simulink model "scheme"  (R2020a)
settings: Solver=VariableStepAuto  StartTime=0.0  StopTime=100  RelTol=1e-3
values from neighbouring files (symbols this model uses):
  G1 = K_r_d.Numerator{1, 1}    [script.m]
  G2 = K_r_d.Denominator{1, 1}    [script.m]
  Ts_ = 0.1    [script.m]
libraries: simulink x1
settings Model: Creator=User  LastModifiedBy=User

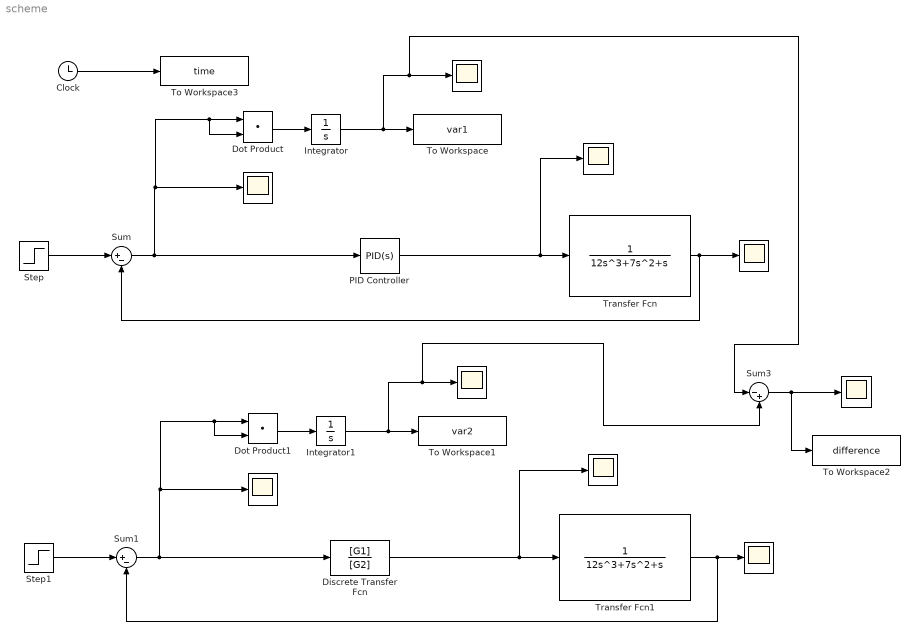
== system scheme ==
  " " : Scope
  "  " : Scope
  "   " : Scope
  "    " : Scope
  "     " : Scope
  "                 " : Scope
  "                       " : Scope
  "                                       " : Scope
  "                                                        " : Scope
  Clock : Clock
  Discrete Transfer Fcn : DiscreteTransferFcn  Numerator=[G1]  Denominator=[G2]  SampleTime=Ts_
  Dot Product : DotProduct  InputSameDT=on  OutDataTypeStr=Inherit: Inherit via internal rule
  Dot Product1 : DotProduct  InputSameDT=on  OutDataTypeStr=Inherit: Inherit via internal rule
  Integrator : Integrator
  Integrator1 : Integrator
  PID Controller : simulink/Continuous/PID Controller  Controller=PID  Form=Parallel  TimeDomain=Continuous-time  UseExternalTs=off  SampleTime=-1  IntegratorMethod=Forward Euler  FilterMethod=Forward Euler  ControllerParametersSource=internal  P=0.2897  I=0.006773  D=2.007  UseFilter=on  N=35.18  TunerSelectOption=Transfer Function Based (PID Tuner App)  InitialConditionSource=internal  InitialConditionForIntegrator=0  InitialConditionForFilter=0  DifferentiatorICPrevScaledInput=0  ExternalReset=none  TrackingMode=off  Kt=1  LimitOutput=off  UpperSaturationLimit=inf  LowerSaturationLimit=-inf  LinearizeAsGain=on  AntiWindupMode=none  Kb=1  POutMin=[]  POutMax=[]  IOutMin=[]  IOutMax=[]  DOutMin=[]  DOutMax=[]  NOutMin=[]  NOutMax=[]  SumOutMin=[]  SumOutMax=[]  SaturationOutMin=[]  SaturationOutMax=[]  PParamMin=[]  PParamMax=[]  IParamMin=[]  IParamMax=[]  DParamMin=[]  DParamMax=[]  NParamMin=[]  NParamMax=[]  KbParamMin=[]  KbParamMax=[]  KtParamMin=[]  KtParamMax=[]  KbOutMin=[]  KbOutMax=[]  KtOutMin=[]  KtOutMax=[]  IntegratorOutMin=[]  IntegratorOutMax=[]  FilterOutMin=[]  FilterOutMax=[]  SumI1OutMin=[]  SumI1OutMax=[]  SumI2OutMin=[]  SumI2OutMax=[]  SumI3OutMin=[]  SumI3OutMax=[]  SumI4OutMin=[]  SumI4OutMax=[]  SumDOutMin=[]  SumDOutMax=[]  DifferentiatorOutMin=[]  DifferentiatorOutMax=[]  FilterDiffOutCoefMin=[]  FilterDiffOutCoefMax=[]  ReciprocalOutMin=[]  ReciprocalOutMax=[]  SumDenOutMin=[]  SumDenOutMax=[]  SumNumOutMin=[]  SumNumOutMax=[]  DivideOutMin=[]  DivideOutMax=[]  UdiffTsProdOutMin=[]  UdiffTsProdOutMax=[]  NTsProdOutMin=[]  NTsProdOutMax=[]  UintegralTsProdOutMin=[]  UintegralTsProdOutMax=[]  UngainTsProdOutMin=[]  UngainTsProdOutMax=[]  IntegratorContinuousStateAttributes=''  IntegratorStateMustResolveToSignalObject=off  IntegratorRTWStateStorageClass=Auto  FilterContinuousStateAttributes=''  FilterStateMustResolveToSignalObject=off  FilterRTWStateStorageClass=Auto  ParallelPVariant=InternalParameters  IdealPVariant=Disabled  IVariant=InternalParameters  DVariant=InternalParameters  IntegratorVariant=Continuous  SatVariant=Disabled  AWVariant=Passthrough  PCopyVariant=Disabled  TRVariant=Disabled  FdbkBlocksVariant=Forward  IdealPFdbkVariant=Disabled  SatFdbkVariant=Disabled  DerivativeFilterVariant=ContFilter  NVariant=InternalParameters  NCopyVariant=Disabled  FilterICVariant=InternalICsFilter  IntegratorICVariant=InternalICs  ExternalResetVariant=Disabled  TRSumVariant=Passthrough  SumFdbkVariant=Disabled  SumVariant=Sum_PID  TsampFilterVariant=InternalTs  TsampNgainVariant=Passthrough  TsampIntegralVariant=Passthrough
  Step : Step  Time=0  SampleTime=0
  Step1 : Step  Time=0  SampleTime=0
  Sum : Sum  Inputs=|+-
  Sum1 : Sum  Inputs=|+-
  Sum3 : Sum  Inputs=|-+
  To Workspace : ToWorkspace  VariableName=var1  SampleTime=-1
  To Workspace1 : ToWorkspace  VariableName=var2  SampleTime=-1
  To Workspace2 : ToWorkspace  VariableName=difference  SampleTime=-1
  To Workspace3 : ToWorkspace  VariableName=time  SampleTime=-1
  Transfer Fcn : TransferFcn  Denominator=[12 7 1 0]
  Transfer Fcn1 : TransferFcn  Denominator=[12 7 1 0]
  wires:
  Transfer Fcn/1 -> Sum/2, "                                                        "/1
  PID Controller/1 -> " "/1, Transfer Fcn/1
  Step/1 -> Sum/1
  Sum/1 -> PID Controller/1, Dot Product/2, Dot Product/1, "                                       "/1
  Integrator/1 -> Sum3/1, "                 "/1, To Workspace/1
  Dot Product/1 -> Integrator/1
  Transfer Fcn1/1 -> Sum1/2, "     "/1
  Sum1/1 -> Discrete Transfer Fcn/1, Dot Product1/2, Dot Product1/1, "   "/1
  Dot Product1/1 -> Integrator1/1
  Step1/1 -> Sum1/1
  Integrator1/1 -> Sum3/2, "  "/1, To Workspace1/1
  Sum3/1 -> "    "/1, To Workspace2/1
  Clock/1 -> To Workspace3/1
  Discrete Transfer Fcn/1 -> "                       "/1, Transfer Fcn1/1
